simulink model "Torque_regulation_and_inverter_simulation_22b"  (R2025b)
settings: Solver=FixedStepAuto  StartTime=0.0  StopTime=10  RelTol=1e-3
undefined symbols (not defined in the file): Ld, Lq, p, psim, tref, Ts, VDC_VECT
libraries: fl_lib x15, nesl_utility x13, ee_lib x4, eeTransforms x2, batteryecm_lib x1, eePmsmCurrentController x1, eePmsmCurrentReferenceGen x1, eePmsmTorqueEstimator x1, eePwmGeneratorTwoLevel x1, eeGeneralControl x1
settings Model: SimulationMode=accelerator  Creator=akame  LastModifiedBy=jungi
settings OptimizationCC: DefaultParameterBehavior=Inlined  UseDivisionForNetSlopeComputation=on  GainParamInheritBuiltInType=on  UseFloatMulNetSlope=on  InlineInvariantSignals=on  PassReuseOutputArgsAs=Individual arguments  ZeroExternalMemoryAtStartup=off  ZeroInternalMemoryAtStartup=off  NoFixptDivByZeroProtection=on  EfficientFloat2IntCast=on  LifeSpan=1  OptimizeBlockOrder=speed  DifferentSizesBufferReuse=on  EfficientTunableParamExpr=on
settings DebuggingCC: ParameterTunabilityLossMsg=error  SFUnexpectedBacktrackingDiag=warning  SFNoUnconditionalDefaultTransitionDiag=warning
settings HardwareCC: ProdBitPerLong=64.0  ProdLongLongMode=on  ProdHWDeviceType=Apple->ARM64
settings SFSimCC: MATLABDynamicMemAlloc=off
settings RTWCC: SystemTargetFile=ert.tlc  TemplateMakefile=ert_default_tmf  GenerateReport=on  BuildConfiguration=Debug  LaunchReport=on  TargetLang=C++  Description=Embedded Coder
settings CodeAppCC: ForceParamTrailComments=on  IgnoreCustomStorageClasses=off  OperatorAnnotations=on  SimulinkDataObjDesc=on  SFDataObjDesc=on  CustomSymbolStrGlobalVar=rt$N$M  CustomSymbolStrType=$N$M  CustomSymbolStrFcn=$N$M$F  CustomSymbolStrMacro=$N$M  InsertBlockDesc=on  EnableCustomComments=on
settings ERTTargetCC: RootIOFormat=Structure reference  ERTCustomFileTemplate=example_file_process.tlc  ERTFilePackagingFormat=CompactWithDataFile  DynamicArrayContainerType=coder::array  TargetLangStandard=C++11 (ISO)  GenerateSampleERTMain=on  IncludeMdlTerminateFcn=off  CombineSignalStateStructs=on  CodeInterfacePackaging=C++ class  SubcomponentCodeInterfacePackaging=C++ class  SupportComplex=off  SupportContinuousTime=on

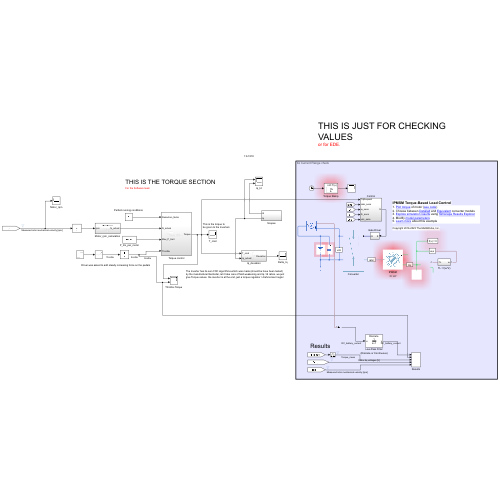
[thumbnail: Simulink's stored preview of the top-level diagram]
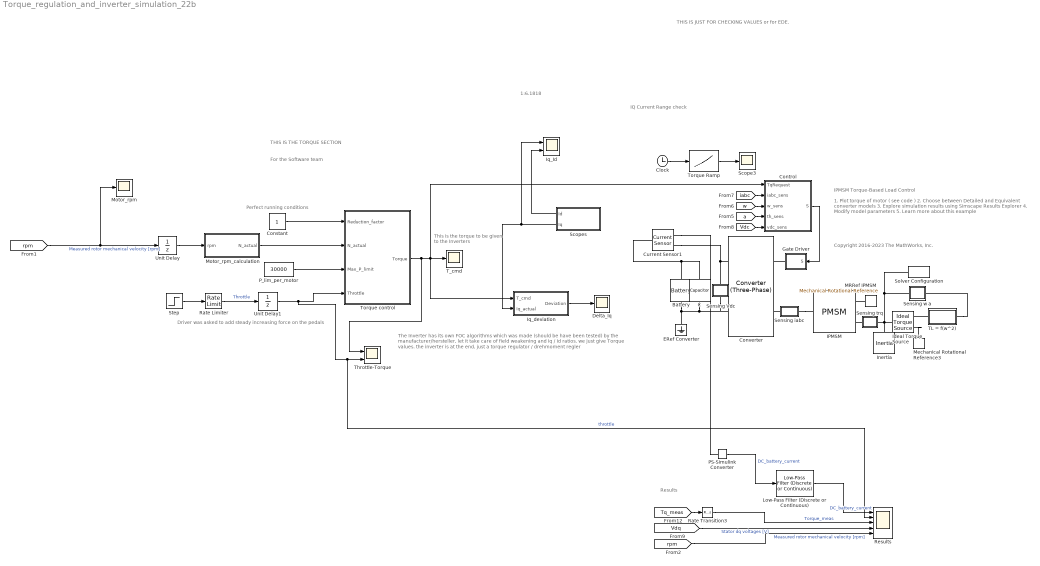
== system Torque_regulation_and_inverter_simulation_22b ==
  note: Results
  note: Perfect running conditions
  note: For the Software team
  note: 1:6.1818
  note: IQ Current Range check
  note: This is the torque to
      | be given to the Inverters
  note: THIS IS JUST FOR CHECKING VALUES
      | or for EDE.
  note: THIS IS THE TORQUE SECTION
  note: Driver was asked to add steady increasing force on the pedals
  note: The Inverter has its own FOC algorithms which was made (should be have been tested) by the manufacturer/hersteller, let it take care of field weakening and Iq / Id ratios. we just give Torque values. the inverter is at the end, just a torque regulator / drehmoment regler
  note: IPMSM Torque-Based Load Control
  note: 1. Plot torque of motor ( see code )
      | 2. Choose between Detailed and Equivalent converter models
      | 3. Explore simulation results using Simscape Results Explorer
      | 4. Modify model parameters
      | 5. Learn more about this example
  note: Copyright 2016-2023 The MathWorks, Inc.
  Battery : batteryecm_lib/Battery  Vnom=Vnom V  prm_dir=1  R1_dis=2 Ohm  R1_ch=2 Ohm  R1=0.001 Ohm  prm_AH=1  AH=10000 hr*A  V1=V1 V  AH1=3000 hr*A  prm_R2=1  R2=2000 Ohm  Tmeas=298.15 K  charge_measurement_port=simscape.enum.battery.enable.no  prm_dyn=1  Rp1=0.005 Ohm  tau1=30 s  Rp2=0.005 Ohm  tau2=30 s  Rp3=0.005 Ohm  tau3=30 s  Rp4=0.005 Ohm  tau4=30 s  Rp5=0.005 Ohm  tau5=30 s  prm_fade=1  N_fade=100  AH_fade=45 hr*A  R1_fade=2.02 Ohm  R1_ch_fade=2.02 Ohm  V1_fade=10.35 V  prm_age=1  prm_age_OCV=1  OCV_age=0.9  SOC_age=60  Tmeas_age=298.15 K  delta_time_age_vec=[0] d  temperature_age_vec=[273] K  OCV_scaling_age=2.2134e6  OCV_offset_age=1.632e6  temp_exp_age=0.515833569 V  t_exp_age=0.75  Vnom_T2=12 V  R1_T2=2.2 Ohm  R1_T2_dis=2.2 Ohm  R1_T2_ch=2.2 Ohm  V1_T2=11.4 V  R2_T2=2200 Ohm  Rp1_T2=0.005 Ohm  tau1_T2=30 s  Rp2_T2=0.005 Ohm  tau2_T2=30 s  Rp3_T2=0.005 Ohm  tau3_T2=30 s  Rp4_T2=0.005 Ohm  tau4_T2=30 s  Rp5_T2=0.005 Ohm  tau5_T2=30 s  Tmeas2=273.15 K  thermal_port=simscape.enum.thermaleffects.omit  thermal_mass=30000 J/K  i_specify=off  i_priority=None  i=0 A  i_nominal_specify=off  i_nominal_value=1  i_nominal_unit=A  v_specify=off  v_priority=None  v=0 V  v_nominal_specify=off  v_nominal_value=1  v_nominal_unit=V  charge_specify=on  charge_priority=High  charge=8000 hr*A  charge_nominal_specify=off  charge_nominal_value=1  charge_nominal_unit=A*hr  num_cycles_specify=off  num_cycles_priority=High  num_cycles=0  num_cycles_nominal_specify=off  num_cycles_nominal_value=1  num_cycles_nominal_unit=1  temperature_specify=off  temperature_priority=High  temperature=298.15 K  temperature_nominal_specify=off  temperature_nominal_value=1  temperature_nominal_unit=K
  C : fl_lib/Electrical/Electrical Elements/Capacitor  c=Cdc uF  r=1e-6 Ohm  g=0 1/Ohm  i_specify=off  i_priority=None  i=0 A  i_nominal_specify=off  i_nominal_value=1  i_nominal_unit=A  v_specify=off  v_priority=None  v=0 V  v_nominal_specify=off  v_nominal_value=1  v_nominal_unit=V  vc_specify=on  vc_priority=None  vc=Vnom V  vc_nominal_specify=off  vc_nominal_value=1  vc_nominal_unit=V
  Clock : Clock
  Constant : Constant
  Control : Subsystem
  Converter : ee_lib/Semiconductors & Converters/Converters/Converter (Three-Phase)  port_option=ee.enum.threePhasePort.composite  fidelity_option=ee.enum.converters.fidelity.detailed  device_type=3  showThermalPort=false  K=0  Vth=0.5 V  Vgt=1 V  Vgt_off=-1 V  Ih=1 A  Vf=0.8 V  Ron=0.001 Ohm  Rds=0.001 Ohm  Goff=1e-5 1/Ohm  Eon_scalar=22.86e-3 J  Eoff_scalar=17.14e-3 J  Eoff_natural_commutation=10e-3 J  Voff=300 V  Iout_scalar=600 A  onCurrentMeasDelay=0 s  useCurrentFromPreviousCycle=false  useVoltageFromPreviousCycle=false  diode_param=2  diode_Vf=0.8 V  diode_Ron=0.001 Ohm  diode_Goff=1e-5 1/Ohm  diode_C=50 nF  diode_iRM=-235 A  diode_iF=300 A  diode_idot=-50 A/us  diode_trr_param=1  diode_trr_factor=3  diode_trr=15 us  diode_Qrr=1.5e+3 s*uA  diode_rec_loss_model=ee.enum.diode.reverseRecoveryModel.fixed  diode_ErecVal=0 J  diode_scaleWithIandV=false  diode_ErecMat=zeros(2, 3) J  diode_TjrecVec=[298.15, 398.15] K  diode_IfrecVec=[.1, 1, 10] A  diode_IrecVal=10 A  diode_VrecVal=10 V  diode_tFilter=1 / 1000 / 100 s  thermal_network_parameterization=ee.enum.thermalNetworkTopology.external  Rth=[.08, .5] K/W  Rth_Cauer=[.08, .1, .5] K/W  Rth_Foster=[.08, .14, .22, .16] K/W  thermal_mass_parameterization=ee.enum.thermalNetwork.timeconstant  thermal_mass=[.01, .5] J/K  thermal_mass_Cauer=[.01, .1, .5] J/K  thermal_mass_Foster=[.001, .005, .05, .5] J/K  thermal_time_constant=[.001, .2] s  thermal_time_constant_Cauer=[.001, .1, .2] s  thermal_time_constant_Foster=[7e-05, .0007, .01, .08] s  thermal_mass_initial_temperatures=[25, 25] degC  thermal_mass_initial_temperatures_Cauer=[25, 25, 25] degC  junction_thermal_mass=0.01 J/K  Tvec_initial_Foster=[25, 25, 25, 25] degC  snubber_type=0  Cs=1e-7 F  Rs=0.1 Ohm  Vce_loss=[0, 150, 300] V
  Current Sensor1 : fl_lib/Electrical/Electrical Sensors/Current Sensor
  Delta_Iq : Scope
      settings: ActiveDisplayYMinimum=-31.0273  ActiveDisplayYMaximum=32.4459  DataLoggingVariableName=ScopeData9
  ERef Converter : fl_lib/Electrical/Electrical Elements/Electrical Reference
  Gate Driver : Subsystem
  IPMSM : ee_lib/Electromechanical/Permanent Magnet/PMSM  port_option=ee.enum.threePhasePort.composite  winding_type=ee.enum.statorconnection.wye  machine_param=ee.enum.pmsm.parameterization.constant  nPolePairs=p  pmflux_param=1  pm_flux_linkage=psim Wb  torque_constant=0.18 N*m/A  back_emf_constant=0.18 V/(rad/s)  stator_param=1  Ld=Ld H  Lq=Lq H  idVec=[-200, 0, 200] A  iqVec=[-200, 0, 200] A  LdMatrix=0.0002 * ones(3, 3) H  LqMatrix=0.0002 * ones(3, 3) H  PmMatrix=0.1 * ones(3, 3) Wb  ktMatrix=0.18 * ones(3, 3) N*m/A  keMatrix=0.18 * ones(3, 3) V/(rad/s)  L0=L0 H  Ls=0.0002 H  Lm=0.00002 H  Ms=0.00002 H  Rs=Rs Ohm  zero_sequence=ee.enum.park.zerosequence.exclude  axes_param=ee.enum.rotorangle.qaxis  loss_param=ee.enum.ironloss.none  losses_oc=[0, 0, 0] W  losses_sc=[0, 0, 0] W  f_losses=60 Hz  Isc_losses=95 A  J=0 kg*m^2  lam=0 N*m/(rad/s)  i_d_specify=off  i_d_priority=None  i_d=0 A  i_d_nominal_specify=off  i_d_nominal_value=1  i_d_nominal_unit=A  i_q_specify=off  i_q_priority=None  i_q=0 A  i_q_nominal_specify=off  i_q_nominal_value=1  i_q_nominal_unit=A  torque_specify=off  torque_priority=None  torque=0 N*m  torque_nominal_specify=off  torque_nominal_value=1  torque_nominal_unit=N*m  angular_velocity_specify=on  angular_velocity_priority=None  angular_velocity=0 rpm  angular_velocity_nominal_specify=off  angular_velocity_nominal_value=1  angular_velocity_nominal_unit=rpm  angular_position_specify=off  angular_position_priority=None  angular_position=0 deg  angular_position_nominal_specify=off  angular_position_nominal_value=1  angular_position_nominal_unit=deg  alpha=3.93e-3 1/K  alpha_flux=-0.001 1/K  Tmeas=298.15 K  stator_thermal_mass=100 J/K  rotor_thermal_mass=200 J/K  Rm_percent_rotor=90  Rd_percent_rotor=30  temperatureA_specify=off  temperatureA_priority=High  temperatureA=25 degC  temperatureA_nominal_specify=off  temperatureA_nominal_value=1  temperatureA_nominal_unit=degC  temperatureB_specify=off  temperatureB_priority=High  temperatureB=25 degC  temperatureB_nominal_specify=off  temperatureB_nominal_value=1  temperatureB_nominal_unit=degC  temperatureC_specify=off  temperatureC_priority=High  temperatureC=25 degC  temperatureC_nominal_specify=off  temperatureC_nominal_value=1  temperatureC_nominal_unit=degC  temperatureR_specify=off  temperatureR_priority=High  temperatureR=25 degC  temperatureR_nominal_specify=off  temperatureR_nominal_value=1  temperatureR_nominal_unit=degC
      settings: AttributesFormatString=35 kW  InternalSimscapePortConfiguration="{\"Bottom\":[],\"Left\":[{\"id\":\"N\",\"label\":\"~\",\"type\":\"foundation.electrical.three_phase\"}],\"Right\":[{\"id\":\"R\",\"label\":\"R\",\"type\":\"foundation.mechanical.rotational.rotational\"},{\"id\":\"C\",\"label\":\"C\",\"type\":\"foundation.mechanical.rotational.rotational\"}],\"Top\":[]}"
  Ideal Torque Source : fl_lib/Mechanical/Mechanical Sources/Ideal Torque Source
  Inertia : fl_lib/Mechanical/Rotational Elements/Inertia  inertia=Jm kg*m^2  num_ports=foundation.enum.numPorts2.one  w_specify=off  w_priority=High  w=0 rad/s  w_nominal_specify=off  w_nominal_value=1  w_nominal_unit=rad/s  t_specify=off  t_priority=None  t=0 N*m  t_nominal_specify=off  t_nominal_value=1  t_nominal_unit=N*m
  Iq_Id : Scope  NumInputPorts=2
      settings: ActiveDisplayYMinimum=-31.1568  ActiveDisplayYMaximum=128.0447  DataLoggingVariableName=ScopeData11
  Iq_deviation : Subsystem
  Low-Pass Filter (Discrete or Continuous) : eeGeneralControl/Low-Pass Filter (Discrete or Continuous)  K=1  T=1  B=inf  A=-inf  init_option=Inherited from block input  x0=0  Ts=-1
  MRRef IPMSM : fl_lib/Mechanical/Rotational Elements/Mechanical Rotational Reference
  Mechanical Rotational Reference3 : fl_lib/Mechanical/Rotational Elements/Mechanical Rotational Reference
  Motor_rpm : Scope
      settings: ActiveDisplayYMinimum=-287.5747  ActiveDisplayYMaximum=2588.1719  DataLoggingVariableName=ScopeData16
  Motor_rpm_calculation : Subsystem
  PS-Simulink Converter : nesl_utility/PS-Simulink Converter  PhysicalDomain=network_engine_domain  SubClassName=ps_output  LeftPortType=input  RightPortType=output  PseudoPeriodic=off  Frequencies=[]  VectorFormat=inherit  Unit=inherit  AffineConversion=off
  P_lim_per_motor : Constant  Value=30000
  Rate Limiter : RateLimiter  SampleTimeMode=inherited
  Rate Transition3 : RateTransition
  Results : Scope  NumInputPorts=5
      settings: ActiveDisplayYMinimum=-3.2765  ActiveDisplayYMaximum=31.5794  DataLoggingVariableName=ScopeData17
  Scope3 : Scope
      settings: ActiveDisplayYMinimum=-1  ActiveDisplayYMaximum=1  DataLoggingVariableName=ScopeData13
  Scopes : Subsystem
      settings: PortSchema="{\"entries\":[{\"content\":{\"sides\":[{\"content\":{\"connectorIds\":[\"Out1\",\"Out2\"]},\"type\":\"ConnectorPlacement.EquallySpacedRectSide\",\"uuid\":\"d68e00e7-054b-4173-9958-dd3b1571d9da\"},{\"content\":{\"side\":\"RIGHT\"},\"type\":\"ConnectorPlacement.EquallySpacedRectSide\",\"uuid\":\"7b48f71f-829e-45e8-b96e-165f80f96185\"},{\"content\":{\"side\":\"TOP\"},\"type\":\"ConnectorPlacement.EquallySpacedRectSide\",\"uuid\":\"a0ffee9d-f8f0-4b9a-8c56-2918da56ae98\"}]},\"type\":\"ConnectorPlacement.EquallySpacedConnector\",\"uuid\":\"f994a5dd-8f07-474a-a565-e3a35d772470\"}],\"packageUris\":[\"http://schema.mathworks.com/mf0/Connector/R2020b\"],\"version\":\"1.0\"}"
  Sensing Vdc : Subsystem
      mask Display: disp('vdc')
  Sensing trq : Subsystem
      mask Display: disp('trq')
  Sensing w a : Subsystem
      mask Display: disp('w,a')
  Sensing iabc : Subsystem
      mask Display: disp('iabc')
  Solver Configuration : nesl_utility/Solver Configuration  PhysicalDomain=network_engine_domain  SubClassName=solver  LeftPortType=input  RightPortType=generic  Tones=[]  Harmonics=[]  SimulateNoise=off  Profile=off  UseLocalSampling=off  EnableSwitchedLinearOptims=on  FrequencyDomain=off  UseCCode=off  RelTol=0.001  AbsTol=1e-06  MinStep=1e-09  ToWorkspace=off  RevertToSquareIcSolve=off  NumHomotopyIterations=100  PhasorMode=off  PhasorModeNumHarmonics=1  ConsistencySolver=NEWTON_FTOL  IndexReductionMethod=DerivativeReplacement  DoDC=off  ResidualTolerance=1e-9  ConsistencyTolSource=GLOBAL  ConsistencyAbsTol=0.001  ConsistencyRelTol=0.001  ConsistencyTolFactor=0.001  UseLocalSolver=on  LocalSolverChoice=NE_BACKWARD_EULER_ADVANCER  ResolveIndetEquations=on  FunctionEvalNumThread=1  LocalSolverSampleTime=Ts  DoFixedCost=on  MaxNonlinIter=5  MaxModeIter=2  ComputeImpulses=off  ImpulseIterations=1  LinearAlgebra=auto  LinearAlgebraNumThread=0  EquationFormulation=NE_TIME_EF  DelaysMemoryBudget=1024  AutomaticFiltering=on  FilteringTimeConstant=0.001  PartitionStorageMethod=AS_NEEDED  PartitionMemoryBudget=1024  PartitionMethod=FAST  MultibodyUseLocalSolver=off  MultibodyLocalSolverChoice=ODE1  MultibodyLocalSolverSampleTime=0.001
  Step : Step  SampleTime=0
  TL = f(w^2) : Subsystem
  T_cmd : Scope
      settings: ActiveDisplayYMinimum=-7.5  ActiveDisplayYMaximum=67.5
  Throttle-Torque : Scope  NumInputPorts=2
      settings: ActiveDisplayYMinimum=-7.4377  ActiveDisplayYMaximum=66.9392  DataLoggingVariableName=ScopeData15
  Torque Ramp : Lookup_n-D  NumberOfTableDimensions=1  BreakpointsForDimension1=[0 0.5 1]  Table=[0 tref tref]  InternalRulePriority=Speed  RndMeth=Simplest
  Torque control : Subsystem
  Unit Delay : UnitDelay  SampleTime=-1  HasFrameUpgradeWarning=on
  Unit Delay1 : UnitDelay  SampleTime=-1  HasFrameUpgradeWarning=on
  wires:
  Constant/1 -> Torque control/1(Reduction_factor)
  Rate Limiter/1 -> Unit Delay1/1  "Throttle"
  P_lim_per_motor/1 -> Torque control/3(Max_P_limit)
  Torque control/1(Torque) -> Throttle-Torque/1, Control/1(TqRequest), Iq_deviation/1(T_cmd), T_cmd/1
  Motor_rpm_calculation/1(N_actual) -> Torque control/2(N_actual)
  Iq_deviation/1(Deviation) -> Delta_Iq/1
  [a] -> Control/4(th_sens)
  Control/1(S) -> Gate Driver/1(S)
  [w] -> Control/3(w_sens)
  [Vdc] -> Control/5(vdc_sens)
  [iabc] -> Control/2(iabc_sens)
  Clock/1 -> Torque Ramp/1
  Scopes/2(Iq) -> Iq_Id/1, Iq_deviation/2(Iq_actual)
  Torque Ramp/1 -> Scope3/1
  [rpm] -> Unit Delay/1, Motor_rpm/1  "Measured rotor mechanical velocity [rpm]"
  Unit Delay/1 -> Motor_rpm_calculation/1(rpm)
  Scopes/1(Id) -> Iq_Id/2
  Rate Transition3/1 -> Results/3  "Torque_meas"
  [Tq_meas] -> Rate Transition3/1
  [Vdq] -> Results/4  "Stator dq voltages [V]"
  [rpm] -> Results/5  "Measured rotor mechanical velocity [rpm]"
  Unit Delay1/1 -> Results/2, Throttle-Torque/2, Torque control/4(Throttle)  "throttle"
  PS-Simulink Converter/1 -> Low-Pass Filter (Discrete or Continuous)/1  "DC_battery_current"
  Low-Pass Filter (Discrete or Continuous)/1 -> Results/1  "DC_battery_current"
  Step/1 -> Rate Limiter/1
  connections:
  Solver Configuration/RConn1 -- Sensing trq/RConn1 -- Ideal Torque Source/LConn1 -- Inertia/LConn1 -- Sensing w a/LConn1
  ERef Converter/LConn1 -- Converter/RConn2 -- Sensing Vdc/RConn1 -- C/RConn1 -- Battery/RConn1
  Battery/LConn1 -- Current Sensor1/LConn1 -- C/LConn1
  TL = f(w^2)/LConn1 -- Sensing w a/RConn1
  Ideal Torque Source/RConn2 -- Mechanical Rotational Reference3/LConn1
  MRRef IPMSM/LConn1 -- IPMSM/RConn2
  Sensing iabc/LConn1 -- Converter/LConn2
  TL = f(w^2)/RConn1 -- Ideal Torque Source/RConn1
  Sensing trq/LConn1 -- IPMSM/RConn1
  Gate Driver/RConn1 -- Converter/LConn1
  Sensing iabc/RConn1 -- IPMSM/LConn1
  Sensing Vdc/LConn1 -- Current Sensor1/RConn2 -- Converter/RConn1
  Current Sensor1/RConn1 -- PS-Simulink Converter/LConn1

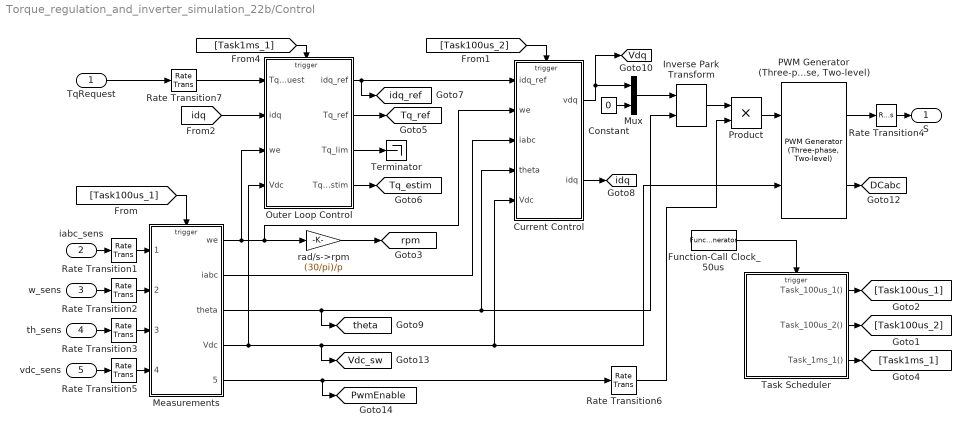
== system Torque_regulation_and_inverter_simulation_22b/Control ==
  TqRequest : Inport
  iabc_sens : Inport  Port=2
  w_sens : Inport  Port=3
  th_sens : Inport  Port=4
  vdc_sens : Inport  Port=5
  Constant : Constant  Value=0  SampleTime=-1
  Current Control : Subsystem
  Function-Call Clock_50us : FunctionCallGenerator  SampleTime=5e-5
  Inverse Park Transform : eeTransforms/Inverse Park Transform  AxisAlignment=Q-axis  PowerInvariant=off
  Measurements : Subsystem
  Mux : Mux  Inputs=2
  Outer Loop Control : Subsystem
  "PWM Generator (Three-phase, Two-level)" : eePwmGeneratorTwoLevel/PWM Generator (Three-phase, Two-level)  PWMMode=Continuous PWM (CPWM)  CPWMMode=SVM: space vector modulation  DPWMMode=60 DPWM: 60 degree discontinuous PWM  fsw=fsw  Ts=Ts
  Product : Product
  Rate Transition{1..7} (7 alike) : RateTransition
  Task Scheduler : Stateflow chart  TreatAsAtomicUnit=on
  Terminator : Terminator
  rad/s->rpm : Gain  Gain=(30/pi)/p
  S : Outport  VectorParamsAs1DForOutWhenUnconnected=off
  tag scope: DCabc=global, PwmEnable=global, Tq_estim=global, Tq_ref=global, Vdc_sw=global, Vdq=global, idq=global, idq_ref=global, rpm=global, theta=global
  wires:
  [Task100us_2] -> Current Control/Trigger
  [Task1ms_1] -> Outer Loop Control/Trigger
  Current Control/1(vdq) -> Mux/1, [Vdq]
  Measurements/2(iabc) -> Current Control/3(iabc)
  Measurements/3(theta) -> [theta], Inverse Park Transform/2, Current Control/4(theta)
  "PWM Generator (Three-phase, Two-level)"/1 -> Rate Transition4/1
  iabc_sens/1 -> Rate Transition1/1
  w_sens/1 -> Rate Transition2/1
  th_sens/1 -> Rate Transition3/1
  vdc_sens/1 -> Rate Transition5/1
  Outer Loop Control/1(idq_ref) -> Current Control/1(idq_ref), [idq_ref]
  "PWM Generator (Three-phase, Two-level)"/2 -> [DCabc]
  Rate Transition1/1 -> Measurements/1(iabc_sens)
  Rate Transition2/1 -> Measurements/2(w_sens)
  Rate Transition3/1 -> Measurements/3(th_sens)
  Rate Transition5/1 -> Measurements/4(Vdc_sens)
  Measurements/4(Vdc) -> Outer Loop Control/4(Vdc), [Vdc_sw], Current Control/5(Vdc), "PWM Generator (Three-phase, Two-level)"/2
  Function-Call Clock_50us/1 -> Task Scheduler/Trigger
  Task Scheduler/3(Task_1ms_1()) -> [Task1ms_1]
  Task Scheduler/2(Task_100us_2()) -> [Task100us_2]
  Task Scheduler/1(Task_100us_1()) -> [Task100us_1]
  Outer Loop Control/2(Tq_ref) -> [Tq_ref]
  Measurements/1(we) -> Outer Loop Control/3(we), Current Control/2(we), rad/s->rpm/1
  rad/s->rpm/1 -> [rpm]
  Outer Loop Control/3(Tq_lim) -> Terminator/1
  Rate Transition7/1 -> Outer Loop Control/1(TqRequest)
  TqRequest/1 -> Rate Transition7/1
  Outer Loop Control/4(Tq_estim) -> [Tq_estim]
  [idq] -> Outer Loop Control/2(idq)
  Rate Transition4/1 -> S/1
  Measurements/5(PwmEnable) -> Rate Transition6/1, [PwmEnable]
  Current Control/2(idq) -> [idq]
  [Task100us_1] -> Measurements/Trigger
  Constant/1 -> Mux/2
  Mux/1 -> Inverse Park Transform/1
  Inverse Park Transform/1 -> Product/1
  Product/1 -> "PWM Generator (Three-phase, Two-level)"/1
  Rate Transition6/1 -> Product/2

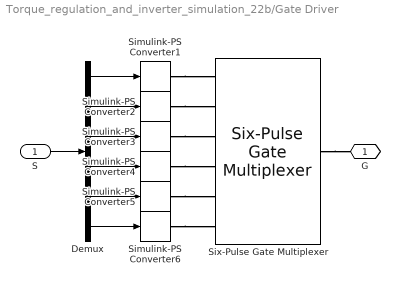
== system Torque_regulation_and_inverter_simulation_22b/Gate Driver ==
  S : Inport
  Demux : Demux  Outputs=6
  Simulink-PS Converter{1..6} (6 alike) : nesl_utility/Simulink-PS Converter  PhysicalDomain=network_engine_domain  SubClassName=ps_input  LeftPortType=input  RightPortType=output  PseudoPeriodic=off  Frequencies=[]  NoiseDistribution=none  NoiseParameters=[]  Unit=1  AffineConversion=off  FilteringAndDerivatives=zero  SimscapeFilterOrder=1  InputFilterTimeConstant=0.001  UdotUserProvided=1
  Six-Pulse Gate Multiplexer : ee_lib/Semiconductors & Converters/Converters/Six-Pulse Gate Multiplexer  port_option=ee.enum.controlport.ps
  G : PMIOPort  Side=Right
  wires:
  Demux/1 -> Simulink-PS Converter1/1
  S/1 -> Demux/1
  Demux/4 -> Simulink-PS Converter4/1
  Demux/2 -> Simulink-PS Converter2/1
  Demux/3 -> Simulink-PS Converter3/1
  Demux/5 -> Simulink-PS Converter5/1
  Demux/6 -> Simulink-PS Converter6/1
  connections:
  Six-Pulse Gate Multiplexer/RConn1 -- G/RConn1
  Simulink-PS Converter1/RConn1 -- Six-Pulse Gate Multiplexer/LConn1
  Simulink-PS Converter3/RConn1 -- Six-Pulse Gate Multiplexer/LConn3
  Simulink-PS Converter5/RConn1 -- Six-Pulse Gate Multiplexer/LConn5
  Simulink-PS Converter6/RConn1 -- Six-Pulse Gate Multiplexer/LConn6
  Simulink-PS Converter4/RConn1 -- Six-Pulse Gate Multiplexer/LConn4
  Simulink-PS Converter2/RConn1 -- Six-Pulse Gate Multiplexer/LConn2

== system Torque_regulation_and_inverter_simulation_22b/Iq_deviation ==
  note: calculate deviation
  note: Iq = Kt / T
  note: Nm/Arms
  T_cmd : Inport
  Iq_actual : Inport  Port=2
  Divide : Product  Inputs=*/
  Kt : Constant  Value=0.54
  Scope : Scope
      settings: ActiveDisplayYMinimum=-1  ActiveDisplayYMaximum=1  DataLoggingVariableName=ScopeData10
  Sum : Sum  Inputs=|+-
  Deviation : Outport
  wires:
  Kt/1 -> Divide/2
  T_cmd/1 -> Divide/1
  Iq_actual/1 -> Scope/1, Sum/1  "iq_actual"
  Divide/1 -> Sum/2  "Calculated_Iq"
  Sum/1 -> Deviation/1

== system Torque_regulation_and_inverter_simulation_22b/Motor_rpm_calculation ==
  note: From CAN Docs Pg 19
      | (Unitek)
  rpm : Inport
  15-Bit_Max_value : Constant  Value=32767
  Constant : Constant  Value=8000
  Divide : Product  Inputs=*/
  Product : Product
  N_actual : Outport
  wires:
  rpm/1 -> Divide/1
  Divide/1 -> Product/1
  15-Bit_Max_value/1 -> Product/2
  Constant/1 -> Divide/2
  Product/1 -> N_actual/1

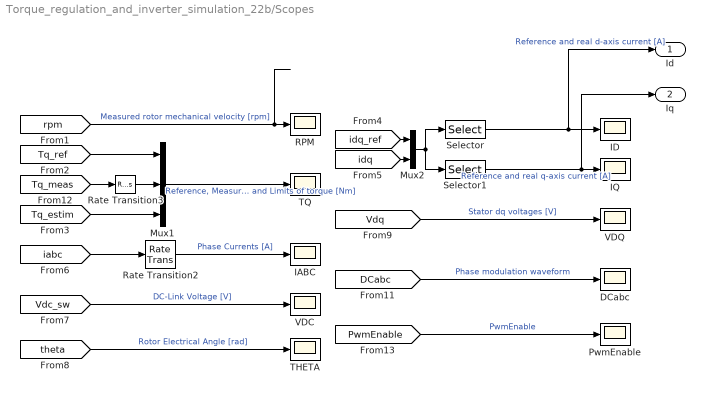
== system Torque_regulation_and_inverter_simulation_22b/Scopes ==
  DCabc : Scope
      settings: ActiveDisplayYMinimum=-1.1466  ActiveDisplayYMaximum=1.1466
  IABC : Scope
      settings: ActiveDisplayYMinimum=-248.4853  ActiveDisplayYMaximum=249.8767  DataLoggingVariableName=ScopeData5
  ID : Scope
      settings: ActiveDisplayYMinimum=-105.3133  ActiveDisplayYMaximum=71.219  DataLoggingSaveFormat=Array
  IQ : Scope
      settings: ActiveDisplayYMinimum=-29.351  ActiveDisplayYMaximum=264.1593  DataLoggingVariableName=ScopeData2  DataLoggingSaveFormat=Array
  Mux1 : Mux  Inputs=3
  Mux2 : Mux  Inputs=2
  PwmEnable : Scope
      settings: ActiveDisplayYMinimum=-0.125  ActiveDisplayYMaximum=1.125  DataLoggingSaveFormat=Array
  RPM : Scope
      settings: ActiveDisplayYMinimum=-354.2074  ActiveDisplayYMaximum=3187.867
  Rate Transition2 : RateTransition  OutPortSampleTime=1e-4
  Rate Transition3 : RateTransition
  Selector : Selector  InputPortWidth=4  IndexOptions=Index vector (dialog)  Indices=[1 3]  OutputSizes=1
  Selector1 : Selector  InputPortWidth=4  IndexOptions=Index vector (dialog)  Indices=[2 4]  OutputSizes=1
  THETA : Scope
      settings: ActiveDisplayYMinimum=-0.78531  ActiveDisplayYMaximum=7.0678  DataLoggingVariableName=ScopeData7
  TQ : Scope
      settings: ActiveDisplayYMinimum=-16.3962  ActiveDisplayYMaximum=123.1336  DataLoggingVariableName=ScopeData2
  VDC : Scope
      settings: ActiveDisplayYMinimum=-51.1546  ActiveDisplayYMaximum=639.2258  DataLoggingVariableName=ScopeData6
  VDQ : Scope
      settings: ActiveDisplayYMinimum=-181.8716  ActiveDisplayYMaximum=95.4205  DataLoggingVariableName=ScopeData8
  Id : Outport
  Iq : Outport  Port=2
  wires:
  [rpm] -> RPM/1  "Measured rotor mechanical velocity [rpm]"
  Mux1/1 -> TQ/1  "Reference, Measured, Estim and Limits of torque [Nm]"
  [Tq_ref] -> Mux1/1
  [iabc] -> Rate Transition2/1
  [theta] -> THETA/1  "Rotor Electrical Angle [rad]"
  [Vdq] -> VDQ/1  "Stator dq voltages [V]"
  [DCabc] -> DCabc/1  "Phase modulation waveform"
  [Vdc_sw] -> VDC/1  "DC-Link Voltage [V]"
  Rate Transition2/1 -> IABC/1  "Phase Currents [A]"
  Selector1/1 -> Iq/1, IQ/1  "Reference and real q-axis current [A]"
  [idq_ref] -> Mux2/1
  Selector/1 -> Id/1, ID/1  "Reference and real d-axis current [A]"
  Mux2/1 -> Selector1/1, Selector/1
  [idq] -> Mux2/2
  [Tq_estim] -> Mux1/3
  [Tq_meas] -> Rate Transition3/1
  Rate Transition3/1 -> Mux1/2
  [PwmEnable] -> PwmEnable/1  "PwmEnable"

== system Torque_regulation_and_inverter_simulation_22b/Sensing Vdc ==
  PS-Simulink Converter4 : nesl_utility/PS-Simulink Converter  PhysicalDomain=network_engine_domain  SubClassName=ps_output  LeftPortType=input  RightPortType=output  PseudoPeriodic=off  Frequencies=[]  VectorFormat=1-D array  Unit=V  AffineConversion=off
  Voltage Sensor : fl_lib/Electrical/Electrical Sensors/Voltage Sensor
  + : PMIOPort  Side=Left
  - : PMIOPort  Port=2  Side=Right
  tag scope: Vdc=global
  wires:
  PS-Simulink Converter4/1 -> [Vdc]
  connections:
  Voltage Sensor/LConn1 -- +/RConn1
  Voltage Sensor/RConn2 -- -/RConn1
  PS-Simulink Converter4/LConn1 -- Voltage Sensor/RConn1

== system Torque_regulation_and_inverter_simulation_22b/Sensing trq ==
  PS-Simulink Converter3 : nesl_utility/PS-Simulink Converter  PhysicalDomain=network_engine_domain  SubClassName=ps_output  LeftPortType=input  RightPortType=output  PseudoPeriodic=off  Frequencies=[]  VectorFormat=1-D array  Unit=N*m  AffineConversion=off
  Torque Sensor : fl_lib/Mechanical/Mechanical Sensors/Ideal Torque Sensor
  R : PMIOPort  Side=Left
  C : PMIOPort  Port=2  Side=Right
  tag scope: Tq_meas=global
  wires:
  PS-Simulink Converter3/1 -> [Tq_meas]
  connections:
  Torque Sensor/RConn1 -- C/RConn1
  Torque Sensor/RConn2 -- PS-Simulink Converter3/LConn1
  Torque Sensor/LConn1 -- R/RConn1

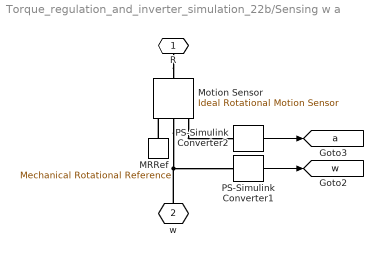
== system Torque_regulation_and_inverter_simulation_22b/Sensing w a ==
  MRRef : fl_lib/Mechanical/Rotational Elements/Mechanical Rotational Reference
  Motion Sensor : fl_lib/Mechanical/Mechanical Sensors/Ideal Rotational Motion Sensor  reference=foundation.enum.MeasurementReference.difference  acceleration_port=false  velocity_port=true  position_port=true  wrap_angle=simscape.enum.onoff.off  offset=0 deg
  PS-Simulink Converter1 : nesl_utility/PS-Simulink Converter  PhysicalDomain=network_engine_domain  SubClassName=ps_output  LeftPortType=input  RightPortType=output  PseudoPeriodic=off  Frequencies=[]  VectorFormat=1-D array  Unit=rad/s  AffineConversion=off
  PS-Simulink Converter2 : nesl_utility/PS-Simulink Converter  PhysicalDomain=network_engine_domain  SubClassName=ps_output  LeftPortType=input  RightPortType=output  PseudoPeriodic=off  Frequencies=[]  VectorFormat=1-D array  Unit=rad  AffineConversion=off
  R : PMIOPort  Side=Left
  w : PMIOPort  Port=2  Side=Right
  tag scope: a=global, w=global
  wires:
  PS-Simulink Converter1/1 -> [w]
  PS-Simulink Converter2/1 -> [a]
  connections:
  R/RConn1 -- Motion Sensor/LConn1
  Motion Sensor/RConn2 -- PS-Simulink Converter1/LConn1 -- w/RConn1
  MRRef/LConn1 -- Motion Sensor/RConn1
  Motion Sensor/RConn3 -- PS-Simulink Converter2/LConn1

== system Torque_regulation_and_inverter_simulation_22b/Sensing iabc ==
  Current Sensor : ee_lib/Sensors & Transducers/Current Sensor (Three-Phase)
  PS-Simulink Converter : nesl_utility/PS-Simulink Converter  PhysicalDomain=network_engine_domain  SubClassName=ps_output  LeftPortType=input  RightPortType=output  PseudoPeriodic=off  Frequencies=[]  VectorFormat=1-D array  Unit=A  AffineConversion=off
  1 : PMIOPort  Side=Left
  2 : PMIOPort  Port=2  Side=Right
  tag scope: iabc=global
  wires:
  PS-Simulink Converter/1 -> [iabc]
  connections:
  1/RConn1 -- Current Sensor/LConn1
  2/RConn1 -- Current Sensor/RConn2
  Current Sensor/RConn1 -- PS-Simulink Converter/LConn1

== system Torque_regulation_and_inverter_simulation_22b/TL = f(w^2) ==
  OG : fl_lib/Physical Signals/Functions/PS Math Function  fcn_choice=7  v=1
  PS Gain : fl_lib/Physical Signals/Functions/PS Gain  gain=1/300 1/(rad/s)
  PS Math Function : fl_lib/Physical Signals/Functions/PS Math Function  fcn_choice=7  v=1
  load_torque : fl_lib/Physical Signals/Functions/PS Gain  gain=-tref N*m
  w : PMIOPort  Side=Left
  TL : PMIOPort  Port=2  Side=Right
  connections:
  load_torque/RConn1 -- TL/RConn1
  load_torque/LConn1 -- PS Math Function/RConn1
  PS Gain/LConn1 -- w/RConn1
  PS Gain/RConn1 -- PS Math Function/LConn1

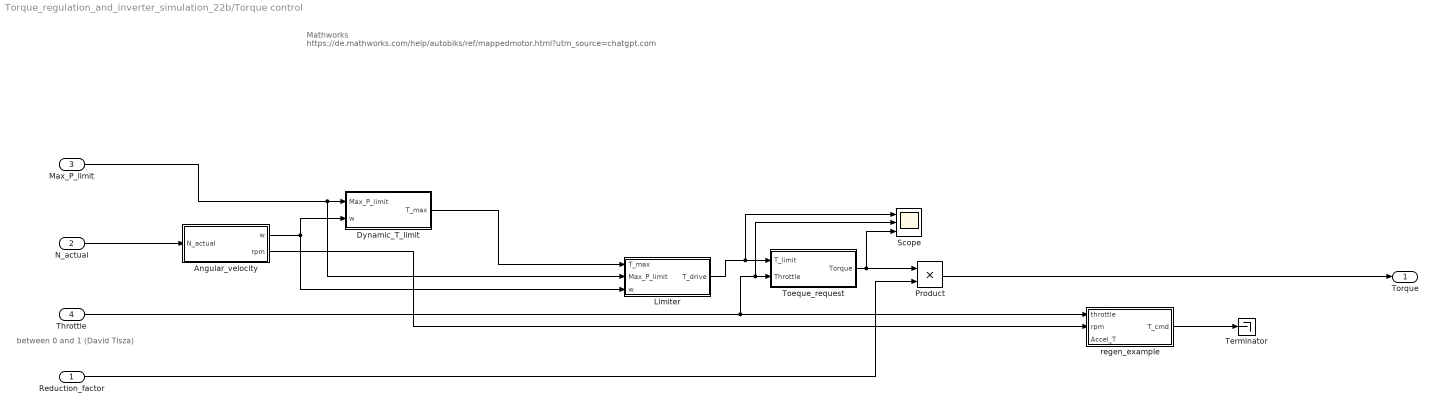
== system Torque_regulation_and_inverter_simulation_22b/Torque control ==
  note: between 0 and 1 (David Tisza)
  note: Mathworks
      | https://de.mathworks.com/help/autoblks/ref/mappedmotor.html?utm_source=chatgpt.com
  Reduction_factor : Inport
  N_actual : Inport  Port=2
  Max_P_limit : Inport  Port=3
  Throttle : Inport  Port=4
  Angular_velocity : Subsystem
  Dynamic_T_limit : Subsystem
  Limiter : Subsystem
  Product : Product
  Scope : Scope  NumInputPorts=3
      settings: ActiveDisplayYMinimum=-13.4845  ActiveDisplayYMaximum=74.4618  DataLoggingVariableName=ScopeData12
  Terminator : Terminator
  Toeque_request : Subsystem
  regen_example : Subsystem
  Torque : Outport
  wires:
  N_actual/1 -> Angular_velocity/1(N_actual)
  Throttle/1 -> regen_example/1(throttle), Scope/2, Toeque_request/2(Throttle)
  Angular_velocity/1(w) -> Limiter/3(w), Dynamic_T_limit/2(w)
  Max_P_limit/1 -> Limiter/2(Max_P_limit), Dynamic_T_limit/1(Max_P_limit)
  Limiter/1(T_drive) -> Scope/1, Toeque_request/1(T_limit)
  Toeque_request/1(Torque) -> Scope/3, Product/1
  Product/1 -> Torque/1
  Reduction_factor/1 -> Product/2
  Dynamic_T_limit/1(T_max) -> Limiter/1(T_max)
  Angular_velocity/2(rpm) -> regen_example/2(rpm)
  regen_example/1(T_cmd) -> Terminator/1

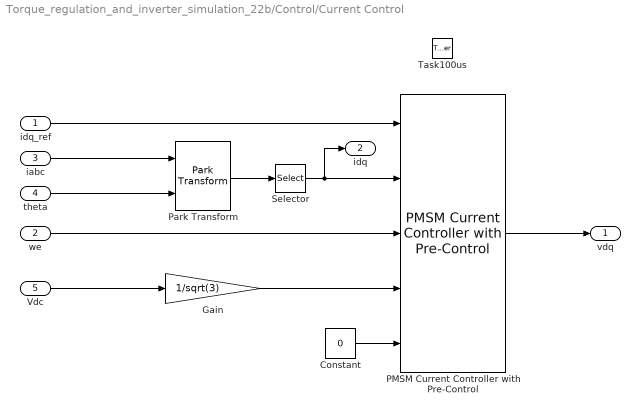
== system Torque_regulation_and_inverter_simulation_22b/Control/Current Control ==
  idq_ref : Inport
  we : Inport  Port=2
  iabc : Inport  Port=3
  theta : Inport  Port=4
  Vdc : Inport  Port=5
  Task100us : TriggerPort  TriggerType=function-call  VariantControl=Variant  PortDimensions=1
  Constant : Constant  Value=0  SampleTime=-1
  Gain : Gain  Gain=1/sqrt(3)
  PMSM Current Controller with Pre-Control : eePmsmCurrentController/PMSM Current Controller with Pre-Control  Kp_id=Kp_id  Ki_id=Ki_id  Kaw_id=1  Kp_iq=Kp_iq  Ki_iq=Ki_iq  Kaw_iq=1  Ts=-1  Tsd=Tsi  AxisPrio=Q-axis  ActZC=on  ActFF=on  idVect=[-200, 0, 200]  iqVect=[-200, 0, 200]  LdMatrix=Ld * ones(3, 3)  LqMatrix=Lq * ones(3, 3)  psimMatrix=psim * ones(3, 3)
  Park Transform : eeTransforms/Park Transform  AxisAlignment=Q-axis  PowerInvariant=off
  Selector : Selector  InputPortWidth=3  IndexOptions=Index vector (dialog)  Indices=[1 2]  OutputSizes=1
  vdq : Outport  VectorParamsAs1DForOutWhenUnconnected=off
  idq : Outport  Port=2  VectorParamsAs1DForOutWhenUnconnected=off
  wires:
  Park Transform/1 -> Selector/1
  Gain/1 -> PMSM Current Controller with Pre-Control/4
  Selector/1 -> idq/1, PMSM Current Controller with Pre-Control/2
  Constant/1 -> PMSM Current Controller with Pre-Control/5
  PMSM Current Controller with Pre-Control/1 -> vdq/1
  we/1 -> PMSM Current Controller with Pre-Control/3
  idq_ref/1 -> PMSM Current Controller with Pre-Control/1
  theta/1 -> Park Transform/2
  iabc/1 -> Park Transform/1
  Vdc/1 -> Gain/1

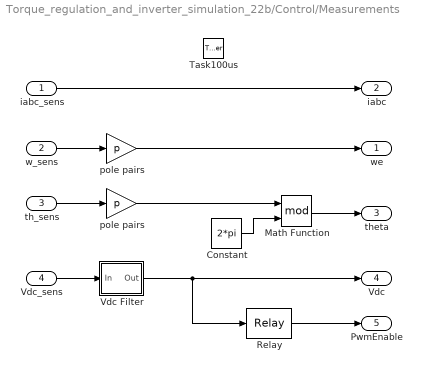
== system Torque_regulation_and_inverter_simulation_22b/Control/Measurements ==
  iabc_sens : Inport
  w_sens : Inport  Port=2
  th_sens : Inport  Port=3
  Vdc_sens : Inport  Port=4
  Task100us : TriggerPort  TriggerType=function-call  VariantControl=Variant  PortDimensions=1
  Constant : Constant  Value=2*pi  SampleTime=-1
  Math Function : Math  Operator=mod  SignedPower=on
  Relay : Relay  OnSwitchValue=VDC_VECT(1)  OffSwitchValue=0.5*VDC_VECT(1)
  Vdc Filter : Subsystem  mask(Discrete first-order filter (Low-pass)){T=0.005, Ts=1e-4}
      mask prompts: T "Time constant (s):"; Ts "Sample time (s):"
      mask help: This block implements a discrete low-pass filter. To calculate the coefficients, the block discretises a continuous low-pass filter using the Tustin method.
      mask init:
      | num = [ Ts/(2*T + Ts), Ts/(2*T + Ts)];
      | den = [ 1, -(2*T - Ts)/(2*T + Ts)];
  pole pairs : Gain  Gain=p
  "pole pairs " : Gain  Gain=p
  we : Outport  VectorParamsAs1DForOutWhenUnconnected=off
  iabc : Outport  Port=2  VectorParamsAs1DForOutWhenUnconnected=off
  theta : Outport  Port=3  VectorParamsAs1DForOutWhenUnconnected=off
  Vdc : Outport  Port=4  VectorParamsAs1DForOutWhenUnconnected=off
  PwmEnable : Outport  Port=5  VectorParamsAs1DForOutWhenUnconnected=off
  wires:
  pole pairs/1 -> we/1
  Vdc_sens/1 -> Vdc Filter/1(In)
  th_sens/1 -> "pole pairs "/1
  w_sens/1 -> pole pairs/1
  iabc_sens/1 -> iabc/1
  "pole pairs "/1 -> Math Function/1
  Constant/1 -> Math Function/2
  Math Function/1 -> theta/1
  Relay/1 -> PwmEnable/1
  Vdc Filter/1(Out) -> Relay/1, Vdc/1

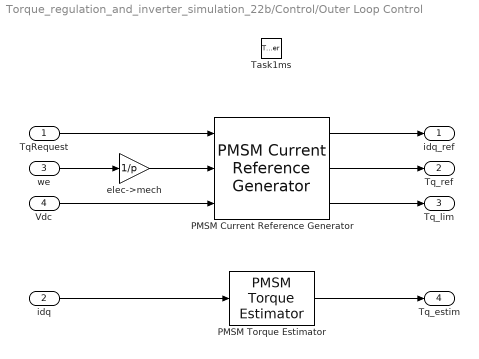
== system Torque_regulation_and_inverter_simulation_22b/Control/Outer Loop Control ==
  TqRequest : Inport
  idq : Inport  Port=2
  we : Inport  Port=3
  Vdc : Inport  Port=4
  Task1ms : TriggerPort  TriggerType=function-call  VariantControl=Variant  PortDimensions=1
  PMSM Current Reference Generator : eePmsmCurrentReferenceGen/PMSM Current Reference Generator  Vnom=Vnom  Pmax=Pmax  Tmax=Tmax  Ts=-1  RefType=Lookup-table based  rpmVec=RPM_VECT  TqVec=TQ_VECT  VdcVec=VDC_VECT  PWMMode=SVM: space vector modulation  ModFactor=1  idMatrix=ID_MAP  iqMatrix=IQ_MAP  p=8  psim=0.04  Ld=0.00024  Lq=0.00029  Rs=0.01  RefExpEnable=0
  PMSM Torque Estimator : eePmsmTorqueEstimator/PMSM Torque Estimator  ParamType=Constant parameters  p=p  idVect=[-200, 200]  iqVect=[-200, 200]  LdMatrix=0.0002 * ones(2, 2)  LqMatrix=0.0002 * ones(2, 2)  psimMatrix=0.04 * ones(2, 2)  Ld=Ld  Lq=Lq  psim=psim  Ts=-1
  elec->mech : Gain  Gain=1/p
  idq_ref : Outport  VectorParamsAs1DForOutWhenUnconnected=off
  Tq_ref : Outport  Port=2  VectorParamsAs1DForOutWhenUnconnected=off
  Tq_lim : Outport  Port=3  VectorParamsAs1DForOutWhenUnconnected=off
  Tq_estim : Outport  Port=4  VectorParamsAs1DForOutWhenUnconnected=off
  wires:
  we/1 -> elec->mech/1
  elec->mech/1 -> PMSM Current Reference Generator/2
  TqRequest/1 -> PMSM Current Reference Generator/1
  Vdc/1 -> PMSM Current Reference Generator/3
  PMSM Current Reference Generator/1 -> idq_ref/1
  PMSM Current Reference Generator/2 -> Tq_ref/1
  PMSM Current Reference Generator/3 -> Tq_lim/1
  idq/1 -> PMSM Torque Estimator/1
  PMSM Torque Estimator/1 -> Tq_estim/1

== system Torque_regulation_and_inverter_simulation_22b/Torque control/Angular_velocity ==
  note: Angular velocity in
      | rad / s
  note: per Minute, therefore / 60
  note: value from Inverter (is not RPM)
  note: well lets say max rpm = 8000 (EMRAX 188 MAX)
  N_actual : Inport
  Constant : Constant  Value=8000
  Gain : Gain  Gain=(2*pi) / 60
  Motor_rpm_calculation : Subsystem
  Scope : Scope  NumInputPorts=2
      settings: ActiveDisplayYMinimum=-140.8461  ActiveDisplayYMaximum=1261.5745
  w : Outport
  rpm : Outport  Port=2
  wires:
  N_actual/1 -> Motor_rpm_calculation/2(N_actual)
  Constant/1 -> Motor_rpm_calculation/1(rpm_max)
  Gain/1 -> Scope/2, w/1  "rad/s"
  Motor_rpm_calculation/1(Motor_rpm) -> rpm/1, Scope/1, Gain/1

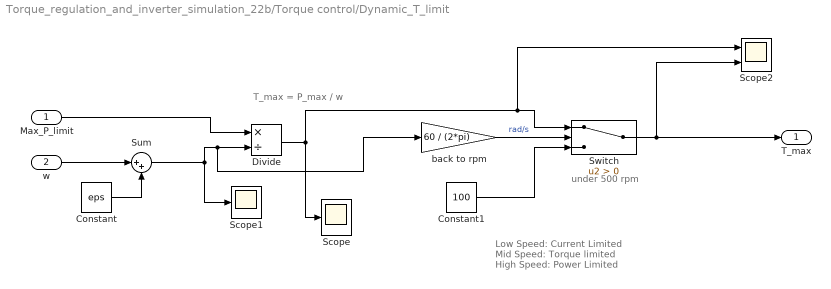
== system Torque_regulation_and_inverter_simulation_22b/Torque control/Dynamic_T_limit ==
  note: under 500 rpm
  note: Low Speed: Current Limited
      | Mid Speed: Torque limited
      | High Speed: Power Limited
  note: T_max = P_max / w
  Max_P_limit : Inport
  w : Inport  Port=2
  Constant : Constant  Value=eps
  Constant1 : Constant  Value=100
  Divide : Product  Inputs=*/
  Scope : Scope
      settings: ActiveDisplayYMinimum=-13932.9318  ActiveDisplayYMaximum=27243.7177  DataLoggingVariableName=ScopeData2
  Scope1 : Scope
      settings: ActiveDisplayYMinimum=-1  ActiveDisplayYMaximum=1  DataLoggingVariableName=ScopeData3
  Scope2 : Scope  NumInputPorts=2
      settings: ActiveDisplayYMinimum=90  ActiveDisplayYMaximum=110  DataLoggingVariableName=ScopeData4
  Sum : Sum  Inputs=|++
  Switch : Switch  Criteria=u2 > Threshold  SaturateOnIntegerOverflow=off  InputSameDT=off
  "back to rpm " : Gain  Gain=60 / (2*pi)
  T_max : Outport
  wires:
  Sum/1 -> Scope1/1, "back to rpm "/1, Divide/2
  Max_P_limit/1 -> Divide/1
  Divide/1 -> Scope/1, Scope2/1, Switch/1
  Constant/1 -> Sum/2
  w/1 -> Sum/1
  Switch/1 -> Scope2/2, T_max/1
  "back to rpm "/1 -> Switch/2  "rad/s"
  Constant1/1 -> Switch/3

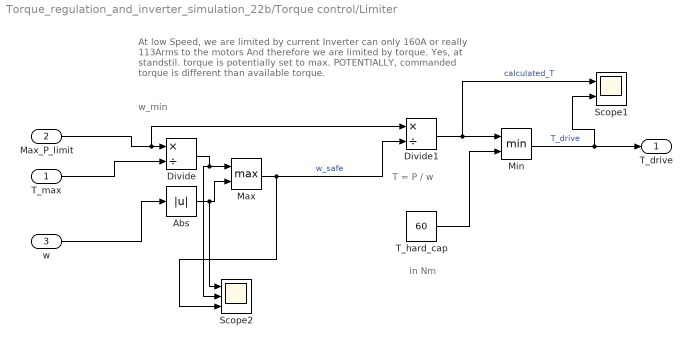
== system Torque_regulation_and_inverter_simulation_22b/Torque control/Limiter ==
  note: T = P / w
  note: in Nm
  note: At low Speed, we are limited by current
      | Inverter can only 160A or really 113Arms to the motors
      |
      | And therefore we are limited by torque.
      | Yes, at standstil. torque is potentially set to max.
      | POTENTIALLY, commanded torque is different than available torque.
  note: w_min
  T_max : Inport
  Max_P_limit : Inport  Port=2
  w : Inport  Port=3
  Abs : Abs  SaturateOnIntegerOverflow=off
  Divide : Product  Inputs=*/
  Divide1 : Product  Inputs=*/
  Max : MinMax  Function=max  Inputs=2
  Min : MinMax  Inputs=2
  Scope1 : Scope  NumInputPorts=2
      settings: ActiveDisplayYMinimum=-1  ActiveDisplayYMaximum=1  DataLoggingVariableName=ScopeData6
  Scope2 : Scope  NumInputPorts=3
      settings: ActiveDisplayYMinimum=-1  ActiveDisplayYMaximum=1  DataLoggingVariableName=ScopeData7
  T_hard_cap : Constant  Value=60
  T_drive : Outport
  wires:
  Max_P_limit/1 -> Divide1/1, Divide/1
  T_max/1 -> Divide/2
  w/1 -> Abs/1
  Divide/1 -> Max/1, Scope2/2
  Abs/1 -> Scope2/1, Max/2
  Max/1 -> Divide1/2, Scope2/3  "w_safe"
  Divide1/1 -> Scope1/1, Min/1  "calculated_T"
  T_hard_cap/1 -> Min/2
  Min/1 -> Scope1/2, T_drive/1  "T_drive"

== system Torque_regulation_and_inverter_simulation_22b/Torque control/Toeque_request ==
  note: T = u * T_max
  note: Between 1 and 0
  T_limit : Inport
  Throttle : Inport  Port=2
  Product : Product
  Saturation : Saturate  UpperLimit=1  LowerLimit=0
  Torque : Outport
  wires:
  Throttle/1 -> Saturation/1
  Saturation/1 -> Product/1
  T_limit/1 -> Product/2
  Product/1 -> Torque/1

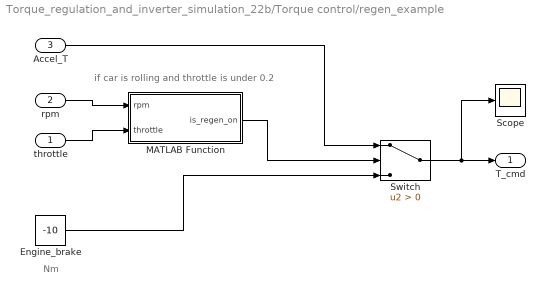
== system Torque_regulation_and_inverter_simulation_22b/Torque control/regen_example ==
  note: if car is rolling and throttle is under 0.2
  note: Nm
  throttle : Inport
  rpm : Inport  Port=2
  Accel_T : Inport  Port=3
  Engine_brake : Constant  Value=-10
  MATLAB Function : MATLAB Function  TreatAsAtomicUnit=on
  Scope : Scope
      settings: ActiveDisplayYMinimum=-11.3023  ActiveDisplayYMaximum=1.7203  DataLoggingVariableName=ScopeData14
  Switch : Switch  Criteria=u2 > Threshold  SaturateOnIntegerOverflow=off  InputSameDT=off
  T_cmd : Outport
  wires:
  Accel_T/1 -> Switch/1
  throttle/1 -> MATLAB Function/2(throttle)
  rpm/1 -> MATLAB Function/1(rpm)
  MATLAB Function/1(is_regen_on) -> Switch/2
  Engine_brake/1 -> Switch/3
  Switch/1 -> Scope/1, T_cmd/1

== system Torque_regulation_and_inverter_simulation_22b/Control/Measurements/Vdc Filter ==
  In : Inport
  Discrete Transfer Fcn : DiscreteTransferFcn  Numerator=num  Denominator=den
  Out : Outport  VectorParamsAs1DForOutWhenUnconnected=off
  wires:
  Discrete Transfer Fcn/1 -> Out/1
  In/1 -> Discrete Transfer Fcn/1

== system Torque_regulation_and_inverter_simulation_22b/Torque control/Angular_velocity/Motor_rpm_calculation ==
  note: From CAN Docs Pg 19
      | (Unitek)
  rpm_max : Inport
  N_actual : Inport  Port=2
  15-Bit_Max_value : Constant  Value=32767
  Divide : Product  Inputs=*/
  Product : Product
  Motor_rpm : Outport
  wires:
  N_actual/1 -> Divide/1
  Divide/1 -> Product/1
  15-Bit_Max_value/1 -> Divide/2
  rpm_max/1 -> Product/2
  Product/1 -> Motor_rpm/1

== stateflow chart Torque_regulation_and_inverter_simulation_22b/Control/Task Scheduler ==
  (default) -> (junction 23) : CLK_50us
  (junction 23) -> (junction 17)
  (junction 17) -> (junction 22) [order 2]
  (junction 17) -> (junction 22) [order 1] : [cnt%%2==0]{Task_100us_1;}
  (junction 22) -> (junction 18) [order 2]
  (junction 22) -> (junction 18) [order 1] : [cnt%%2==0]{Task_100us_2;}
  (junction 18) -> (junction 21) [order 1] : [cnt%%20==0]{Task_1ms_1;}
  (junction 18) -> (junction 21) [order 2]
  (junction 21) -> (junction 34) [order 2]
  (junction 21) -> (junction 16) [order 1] : [1]{cnt++;}
  data: cnt local int32
  events: Task_100us_1 output FUNCTION_CALL_EVENT; Task_100us_2 output FUNCTION_CALL_EVENT; Task_1ms_1 output FUNCTION_CALL_EVENT; CLK_50us input FUNCTION_CALL_EVENT

== matlab function Torque_regulation_and_inverter_simulation_22b/Torque control/regen_example/MATLAB Function ==
  data: rpm input; is_regen_on output; throttle input
function is_regen_on = fcn(rpm, throttle)

if (rpm > 0 && throttle < 0.2)
    is_regen_on = 1;
else
    is_regen_on = 0;
end
